simulink model "SimToTF"  (R2022b)
settings: Solver=VariableStepAuto  StartTime=0.0  StopTime=700  RelTol=1e-3
settings Model: Creator=user  LastModifiedBy=user

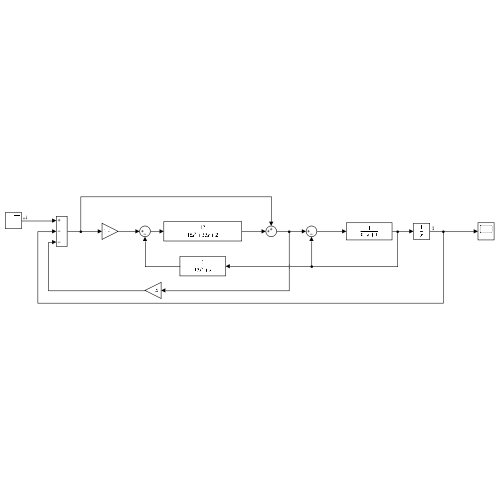
[thumbnail: Simulink's stored preview of the top-level diagram]
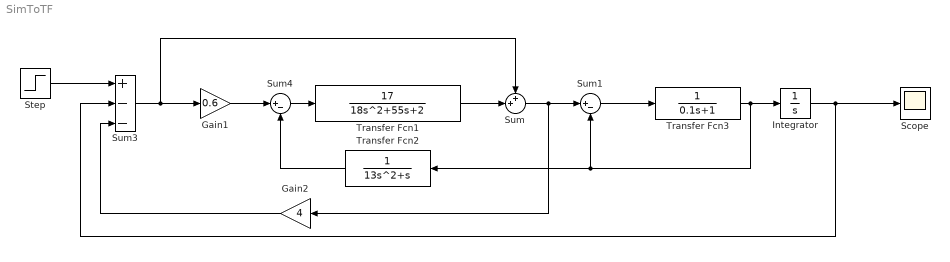
== system SimToTF ==
  Gain1 : Gain  Gain=0.6
  Gain2 : Gain  Gain=4
  Integrator : Integrator
  Scope : Scope
  Step : Step  SampleTime=0
  Sum : Sum  Inputs=++|
  Sum1 : Sum  Inputs=|+-
  Sum3 : Sum  Inputs=+--
  Sum4 : Sum  Inputs=|+-
  Transfer Fcn1 : TransferFcn  Numerator=[17]  Denominator=[18 55 2]
  Transfer Fcn2 : TransferFcn  Denominator=[13 1 0]
  Transfer Fcn3 : TransferFcn  Denominator=[0.1 1]
  wires:
  Step/1 -> Sum3/1
  Transfer Fcn1/1 -> Sum/2
  Sum3/1 -> Gain1/1, Sum/1
  Transfer Fcn3/1 -> Integrator/1, Transfer Fcn2/1, Sum1/2
  Sum4/1 -> Transfer Fcn1/1
  Transfer Fcn2/1 -> Sum4/2
  Gain1/1 -> Sum4/1
  Integrator/1 -> Scope/1, Sum3/2
  Sum1/1 -> Transfer Fcn3/1
  Sum/1 -> Gain2/1, Sum1/1
  Gain2/1 -> Sum3/3
